simulink model "Load_Simulation_08"  (R2017a)
settings: Solver=ode23tb  StartTime=0.0  StopTime=3600  MaxStep=0.1  RelTol=1e-4  EnableMultiTasking=on
undefined symbols (not defined in the file or in its folder): Acid, Hydride, Ion, Lead, Lithium, Metal, Nickel
libraries: powerlib x4, electricdrivelib x3
Description:
  | Copyright 2008-2017 The MathWorks, Inc.
settings Model: SimulationMode=accelerator  Creator=MathWorks  LastModifiedBy=hlope
settings DataIOCC: SaveFormat=Array  SignalLoggingSaveFormat=ModelDataLogs  SignalLogging=off  DSMLogging=off  ReturnWorkspaceOutputs=on  OutputSaveName=V1,V2,V3,S1,S2,S3  ReturnWorkspaceOutputsName=V1,V2,V3,S1,S2,S3
settings OptimizationCC: ExpressionDepthLimit=2147483647  InitFltsAndDblsToZero=on  LifeSpan=inf
settings DebuggingCC: UnderspecifiedInitializationDetection=Classic  MergeDetectMultiDrivingBlocksExec=none  SignalResolutionControl=TryResolveAllWithWarning  SolverPrmCheckMsg=warning  FcnCallInpInsideContextMsg=warning  AllowSymbolicDim=off  StateNameClashWarn=warning  SFUnexpectedBacktrackingDiag=warning  SFNoUnconditionalDefaultTransitionDiag=warning  SFExecutionAtInitializationDiag=none
settings HardwareCC: ProdBitPerPointer=32  ProdBitPerSizeT=32  ProdBitPerPtrDiffT=32  ProdLargestAtomicFloat=None  ProdIntDivRoundTo=Undefined  ProdEndianess=Unspecified  ProdWordSize=32  ProdHWDeviceType=32-bit Generic
settings ModelReferenceCC: PropagateSignalLabelsOutOfModel=off
settings GRTTargetCC: TargetLangStandard=C89/C90 (ANSI)  GeneratePreprocessorConditionals=Disable all  CombineOutputUpdateFcns=off  GRTInterface=on
settings ConfigComp: CovMetricSettings=dw  CovHtmlReporting=on  CovSaveCumulativeToWorkspaceVar=on  CovSaveSingleToWorkspaceVar=on  CovExternalEMLEnable=off

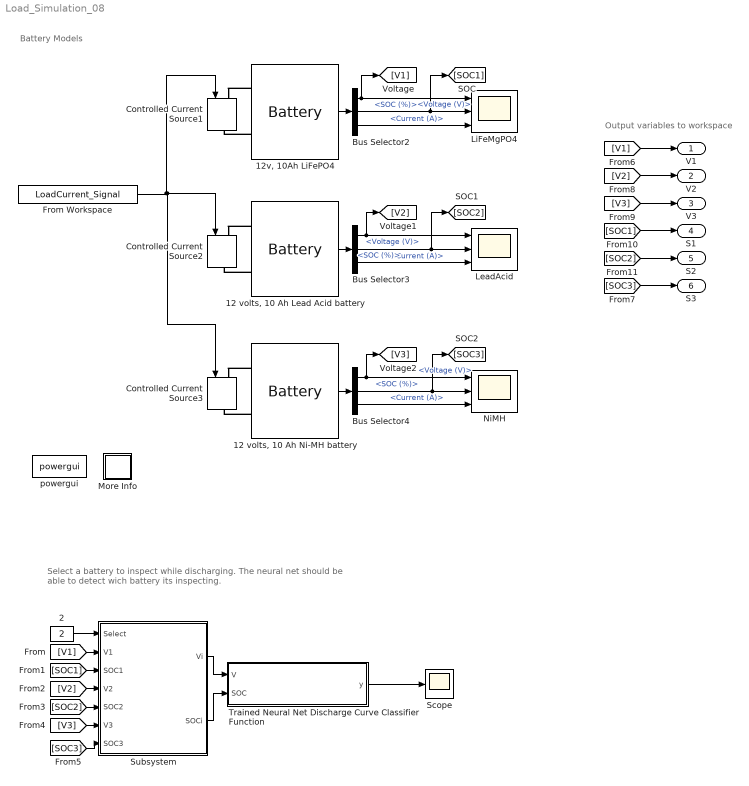
== system Load_Simulation_08 ==
  note: Output variables to workspace
  note: Select a battery to inspect while discharging.
      | The neural net should be able to detect wich battery its inspecting.
  note: Battery Models
  " 2" : Constant  Value=2
  "12 volts, 10 Ah Lead Acid battery " : electricdrivelib/Extra Sources/Battery  BatType=Lead-Acid  ShowTempParam=on  ThermalPreset=no  ShowAgeParam=off  NomV=24  NomQ=10  SOC=100  Batt_Tr=30  PresetModel=on  MaxQ=10.4167  MinV=18  FullV=26.1316  Dis_rate=2  R=0.024  Normal_OP=3.1028  expZone="[24.4342    0.0333333]"  current=[1,5,10,15,20]  Units=Ampere-hour  Tci=20  NomT=25  T2=0  MaxQ2=2.208  FullV2=3.45  Normal_OP2=2.8  expZone2="[3.22        0.23]"  Rca=0.6  ti=1000  Dp=0  Neq0=0  Tsim=1e6  Ta1=25  Qeol=5.4*0.9  Reol=0.013333*1.2  Char_age=[2.3478, 3]  Dis_age=[2.3478, 10]  N1=1500  N2=10500  N3=1000  N4=1400  Ta2=45  N5=950
  "12 volts, 10 Ah Ni-MH battery" : electricdrivelib/Extra Sources/Battery  BatType=Nickel-Metal-Hydride  ShowTempParam=on  ThermalPreset=no  ShowAgeParam=off  NomV=24  NomQ=10  SOC=100  Batt_Tr=30  PresetModel=on  MaxQ=10.7692  MinV=18  FullV=28.2712  Dis_rate=2  R=0.024  Normal_OP=9.6154  expZone="[26.0339            2]"  current=[1,5,10,15,20]  Units=Ampere-hour  Tci=20  NomT=25  T2=0  MaxQ2=2.208  FullV2=3.45  Normal_OP2=2.8  expZone2="[3.22        0.23]"  Rca=0.6  ti=1000  Dp=0  Neq0=0  Tsim=1e6  Ta1=25  Qeol=5.4*0.9  Reol=0.013333*1.2  Char_age=[2.3478, 3]  Dis_age=[2.3478, 10]  N1=1500  N2=10500  N3=1000  N4=1400  Ta2=45  N5=950
  "12v, 10Ah LiFePO4 " : electricdrivelib/Extra Sources/Battery  BatType=Lithium-Ion  ShowTempParam=off  ThermalPreset="12.8V  40Ah  (LiFeMgPO4)"  ShowAgeParam=off  NomV=24  NomQ=10  SOC=100  Batt_Tr=30  PresetModel=off  MaxQ=10  MinV=18  FullV=13.9678  Dis_rate=2  R=0.012  Normal_OP=9.0435  expZone="[12.9646     0.491304]"  current=[1,5,10,15,20]  Units=Time  Tci=20  NomT=20  T2=0  MaxQ2=36  FullV2=13  Normal_OP2=11.7  expZone2="[12.67            4]"  Rca=0.6411  ti=4880  Dp=0  Neq0=0  Tsim=1e6  Ta1=25  Qeol=5.4*0.9  Reol=0.013333*1.2  Char_age=[2.3478, 3]  Dis_age=[2.3478, 10]  N1=1500  N2=10500  N3=1000  N4=1400  Ta2=45  N5=950
  Bus Selector2 : BusSelector  OutputSignals=Voltage (V),SOC (%),Current (A)
  Bus Selector3 : BusSelector  OutputSignals=Voltage (V),SOC (%),Current (A)
  Bus Selector4 : BusSelector  OutputSignals=Voltage (V),SOC (%),Current (A)
  Controlled Current Source1 : powerlib/Electrical Sources/Controlled Current Source  Initialize=on  Source_Type=AC  Amplitude=0  Phase=0  Frequency=0  Measurements=None
  Controlled Current Source2 : powerlib/Electrical Sources/Controlled Current Source  Initialize=on  Source_Type=AC  Amplitude=0  Phase=0  Frequency=0  Measurements=None
  Controlled Current Source3 : powerlib/Electrical Sources/Controlled Current Source  Initialize=on  Source_Type=AC  Amplitude=0  Phase=0  Frequency=0  Measurements=None
  From Workspace : FromWorkspace  VariableName=LoadCurrent_Signal  SampleTime=0
  LeadAcid : Scope  NumInputPorts=3
  LiFeMgPO4 : Scope  NumInputPorts=3
  More Info : Subsystem
      settings: OpenFcn=showdemo(bdroot(gcb))
      mask Display: disp('?')
  NiMH : Scope  NumInputPorts=3
  Scope : Scope
  Subsystem : Subsystem
  Trained Neural Net Discharge Curve Classifier Function : MATLAB Function  TreatAsAtomicUnit=on
  powergui : powerlib/powergui  SimulationMode=Continuous  SampleTime=0.001  frequency=60  Iterations=50  frequencyindice=0  Pbase=100e6  ErrMax=1e-4  UnitsV=kV  UnitsW=MW  buscounter=0  FunctionMessages=off  echomessages=off  EnableUseOfTLC=off  CurrentSourceSwitches=off  DisableSnubberDevices=off  DisableRonSwitches=off  DisableVfSwitches=off  DisplayEquations=off  SolverType=Tustin  Interpol=off  ExternalGateDelay=off  methode=off  Ts=0  x0status=blocks  SPID=off  SwTol=0  HookPort=off  RestoreLinks=warning  ResistiveCurrentMeasurement=off  Frange=[0:2:500]  Ylog=off  Xlog=on  ShowGrid=off  save=off  variable=ZData  structure=0  ZoomFFT=on  StartTime=0.0  cycles=1  DisplayStyle=1  fundamental=60  FreqAxis=off  MaxFrequency=1000  frequencyindicesteady=1  RmsSteady=1  display=off
  V1 : Outport
  V2 : Outport  Port=2
  V3 : Outport  Port=3
  S1 : Outport  Port=4
  S2 : Outport  Port=5
  S3 : Outport  Port=6
  wires:
  "12 volts, 10 Ah Ni-MH battery"/1 -> Bus Selector4/1
  Bus Selector3/3 -> LeadAcid/3  "<Current (A)>"
  Bus Selector4/3 -> NiMH/3  "<Current (A)>"
  Bus Selector3/1 -> LeadAcid/1, [V2]  "<Voltage (V)>"
  "12v, 10Ah LiFePO4 "/1 -> Bus Selector2/1
  Bus Selector3/2 -> [SOC2], LeadAcid/2  "<SOC (%)>"
  Bus Selector4/2 -> [SOC3], NiMH/2  "<SOC (%)>"
  Bus Selector4/1 -> NiMH/1, [V3]  "<Voltage (V)>"
  Bus Selector2/2 -> LiFeMgPO4/2, [SOC1]  "<SOC (%)>"
  Bus Selector2/1 -> LiFeMgPO4/1, [V1]  "<Voltage (V)>"
  Bus Selector2/3 -> LiFeMgPO4/3  "<Current (A)>"
  "12 volts, 10 Ah Lead Acid battery "/1 -> Bus Selector3/1
  Trained Neural Net Discharge Curve Classifier Function/1(y) -> Scope/1
  From Workspace/1 -> Controlled Current Source1/1, Controlled Current Source3/1, Controlled Current Source2/1
  " 2"/1 -> Subsystem/1(Select)
  Subsystem/1(Vi) -> Trained Neural Net Discharge Curve Classifier Function/1(V)
  Subsystem/2(SOCi) -> Trained Neural Net Discharge Curve Classifier Function/2(SOC)
  [V1] -> Subsystem/2(V1)
  [SOC1] -> Subsystem/3(SOC1)
  [V2] -> Subsystem/4(V2)
  [SOC2] -> Subsystem/5(SOC2)
  [V3] -> Subsystem/6(V3)
  [SOC3] -> Subsystem/7(SOC3)
  [V1] -> V1/1
  [V2] -> V2/1
  [V3] -> V3/1
  [SOC1] -> S1/1
  [SOC2] -> S2/1
  [SOC3] -> S3/1
  connections:
  "12v, 10Ah LiFePO4 "/LConn2 -- Controlled Current Source1/RConn1
  "12 volts, 10 Ah Lead Acid battery "/LConn1 -- Controlled Current Source2/LConn1
  "12 volts, 10 Ah Ni-MH battery"/LConn2 -- Controlled Current Source3/RConn1
  "12 volts, 10 Ah Ni-MH battery"/LConn1 -- Controlled Current Source3/LConn1
  "12 volts, 10 Ah Lead Acid battery "/LConn2 -- Controlled Current Source2/RConn1
  "12v, 10Ah LiFePO4 "/LConn1 -- Controlled Current Source1/LConn1

== system Load_Simulation_08/More Info ==

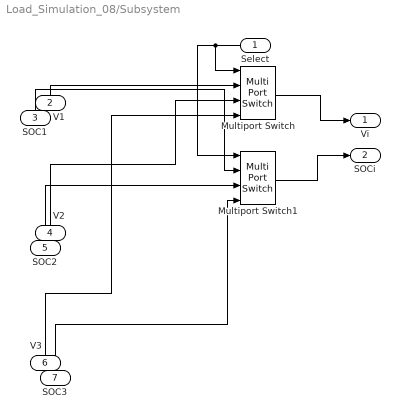
== system Load_Simulation_08/Subsystem ==
  Select : Inport
  V1 : Inport  Port=2
  SOC1 : Inport  Port=3
  V2 : Inport  Port=4
  SOC2 : Inport  Port=5
  V3 : Inport  Port=6
  SOC3 : Inport  Port=7
  Multiport Switch : MultiPortSwitch
  Multiport Switch1 : MultiPortSwitch
  Vi : Outport
  SOCi : Outport  Port=2
  wires:
  Multiport Switch/1 -> Vi/1
  Select/1 -> Multiport Switch1/1, Multiport Switch/1
  Multiport Switch1/1 -> SOCi/1
  V3/1 -> Multiport Switch/4
  SOC2/1 -> Multiport Switch1/3
  SOC1/1 -> Multiport Switch1/2
  SOC3/1 -> Multiport Switch1/4
  V1/1 -> Multiport Switch/2
  V2/1 -> Multiport Switch/3

== matlab function Load_Simulation_08/Trained Neural Net Discharge Curve Classifier Function ==
  data: V input; SOC input; y output
function y = fcn(V,SOC)

x1=[SOC,V];
o = Battery_Classifier(x1);
pcnt = mean(o.')';
[m,i]= max(pcnt);
y= i;
